simulink model "Heating_Six_Rooms_LQG"  (R2023a)
settings: Solver=VariableStepAuto  StartTime=0.0  StopTime=800  RelTol=1e-3
undefined symbols (not defined in the file): A, B, C, Continuous, D, K2, R, Time
libraries: simulink x2, ctrlSharedLib x1
settings Model: Creator=logan  LastModifiedBy=oluwafemiajeigbe
settings OptimizationCC: ReuseModelBlockBuffer=off

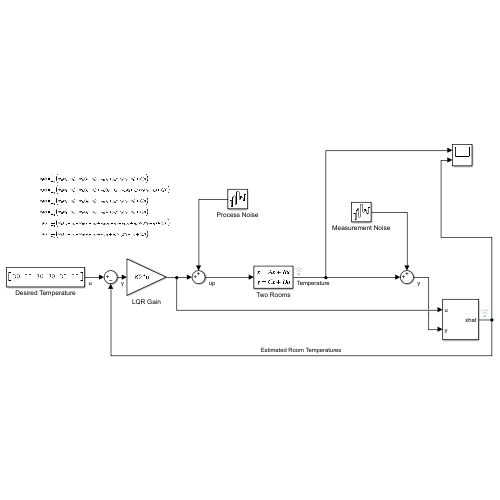
[thumbnail: Simulink's stored preview of the top-level diagram]
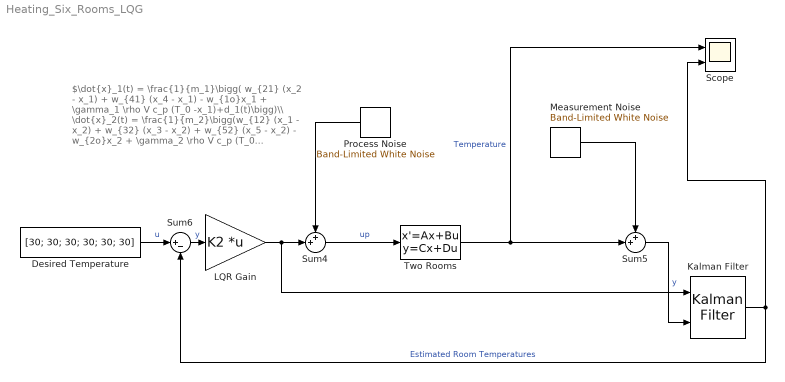
== system Heating_Six_Rooms_LQG ==
  note: $\dot{x}_1(t) = \frac{1}{m_1}\bigg( w_{21} (x_2 - x_1) + w_{41} (x_4 - x_1) - w_{1o}x_1 + \gamma_1 \rho V c_p (T_0 -x_1)+d_1(t)\bigg)\\ \dot{x}_2(t) = \frac{1}{m_2}\bigg(w_{12} (x_1 - x_2) + w_{32} (x_3 - x_2) + w_{52} (x_5 - x_2) - w_{2o}x_2 + \gamma_2 \rho V c_p (T_0 -x_2)+d_2(t)\bigg)\\ \dot{x}_3(t) = \frac{1}{m_3}\bigg( w_{23} (x_2 - x_3) + w_{63} (x_6 - x_3) - w_{3o}x_3 + \gamma_3 \rho V c_p (T_0 -x_3)+d_3(t)\bigg)\\ \dot{x}_4(t) = \frac{1}{m_4}\bigg( w_{14} (x_1 - x_4) + w_{54} (x_5 - x_4) - w_{4o}x_4 + \gamma_4 \rho V c_p (T_0 -x_4)+d_4(t)\bigg)\\ \dot{x}_5(t) = \frac{1}{m_5}\bigg( w_{25} (x_2 - x_5) + w_{45} (x_4 - x_5) + w_{65} (x_6 - x_5) - w_{5o}x_5 + \gamma_5 \rho V c_p (T_0 -x_5)+d_5(t)\bigg)\\ \dot{x}_6(t) = \frac{1}{m_6}\bigg(w_{36} (x_3 - x_6) + w_{56} (x_5 - x_6) - w_{6o}x_6 + \gamma_6 \rho V c_p (T_0 -x_6)+d_6(t)\bigg)$
  Desired Temperature : Constant  Value=[30; 30; 30; 30; 30; 30]
  Kalman Filter : ctrlSharedLib/Kalman Filter  TimeDomain=Continuous-Time  UseCurrentEstimator=on  ModelSource=Individual A, B, C, D matrices  ModelSourceVariable=Plant  A=A  B=B  C=C  D=D  NumberOfStates=1  NumberOfInputs=1  NumberOfOutputs=1  InitialEstimateSource=Dialog  X0=15  P0=10  UseK=off  UseGH=on  NumberOfProcessNoiseInputs=1  G=G  TimeInvariantG=on  H=0  TimeInvariantH=on  Q=Q  TimeInvariantQ=on  R=R  TimeInvariantR=on  N=0  TimeInvariantN=on  AddInputPort=on  AddEnablePort=off  OutputEstimatedY=off  OutputP=off  Ts=-1
  LQR Gain : Gain  Gain=K2  Multiplication=Matrix(K*u)
  Measurement Noise : simulink/Sources/Band-Limited White Noise  Cov=[0 0 0 0 0 0]  Ts=0.1  seed=[23341]
  Process Noise : simulink/Sources/Band-Limited White Noise  Cov=[0 0 0 0 0 0]  Ts=0.1  seed=[23341]
  Scope : Scope  NumInputPorts=2
  Sum4 : Sum  Inputs=++|
  Sum5 : Sum  Inputs=++|
  Sum6 : Sum  Inputs=|+-
  Two Rooms : StateSpace  A=A  B=B  C=C  D=D  InitialCondition=15
  wires:
  Kalman Filter/1 -> Scope/2, Sum6/2  "Estimated Room Temperatures"
  Desired Temperature/1 -> Sum6/1  "u"
  Sum6/1 -> LQR Gain/1  "y"
  LQR Gain/1 -> Kalman Filter/1, Sum4/2
  Process Noise/1 -> Sum4/1
  Sum4/1 -> Two Rooms/1  "up"
  Two Rooms/1 -> Sum5/2, Scope/1  "Temperature"
  Sum5/1 -> Kalman Filter/2  "y"
  Measurement Noise/1 -> Sum5/1
